simulink model "f16_hifi_euler_vTrim"  (R2020b)
settings: Solver=ode4  StartTime=0.0  StopTime=simTime  FixedStep=stepTime  RelTol=1e-3
undefined symbols (not defined in the file): data, ft, outputs, s
libraries: libAeroLookUpTables x9, aerolibconvert2 x7, lib6DOFUtilityEquations x6, libTFActuatorCalc x5, aerolibtransform2 x1, libEngineAngMomSpecs x1, libAircraftMoISpecs x1, libAircraftWeightandMassSpec x1, libAircraftWingFusalageSpecs x1, libCmdPowConversion x1, libEngineThrustCalc x1, libAtmosphereModel x1
(part 1 of 3)
settings Model: Creator=caatay  LastModifiedBy=caatay
settings DataIOCC: SaveOutput=off  SignalLogging=off  DSMLogging=off  ReturnWorkspaceOutputsName=F16_HiFi_vTrim

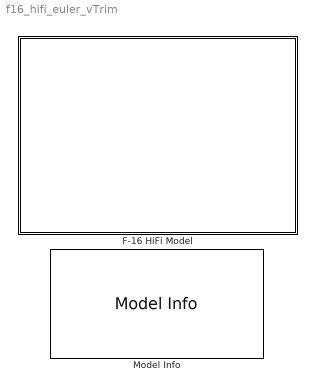
== system f16_hifi_euler_vTrim ==
  F-16 HiFi Model : Subsystem
      mask Display: image('f16-main.jpg'); % Use "Edit Image" on toolstrip to change.
  Model Info : simulink/Model-Wide Utilities/Model Info  Frame=on  DisplayStringWithTags=|  HorizontalTextAlignment=Center  LeftAlignmentValue=0.5
      | High Fidelity F-16 Just Trim Model v%<ModelVersion>
      | -------------------------------------------------------
      | Created By:  %<Creator>
      | Created at:  %<Created>
      | -------------------------------------------------------
      | Modified By: %<LastModifiedBy>
      | Modified at:  %<LastModificationDate>
      | -------------------------------------------------------

== system f16_hifi_euler_vTrim/F-16 HiFi Model ==
  Actuator Model : Subsystem
      mask Display: image('f16-actuator2.jpg'); % Use "Edit Image" on toolstrip to change.
  Aerodynamic Model : Subsystem
      mask Display: image('f16-aerodynamic.jpg'); % Use "Edit Image" on toolstrip to change.
  Aircraft Specifications : Subsystem
      mask Display: image('f16-aircraftSpec.png'); % Use "Edit Image" on toolstrip to change.
  Engine Model : Subsystem
      mask Display: image('f16-engine.jpg'); % Use "Edit Image" on toolstrip to change.
  Environment Model : Subsystem
      mask Display: image('atmosphere.jpg'); % Use "Edit Image" on toolstrip to change.
  Equation of Motion : Subsystem
      mask Display: image('f16-eom.png'); % Use "Edit Image" on toolstrip to change.
  Flight Control System & Cockpit : Subsystem
      mask Display: image('f16-cockpit.jpg'); % Use "Edit Image" on toolstrip to change.
  FlightGear Animation : libFlightGearAnimation/FlightGear Animation  Commented=on  stepTime=stepTime  mask(Animation Model - Flight Gear Animation Model){}
      mask Display: image('flightGear-logo.png'); % Use "Edit Image" on toolstrip to change.
  wires:
  Flight Control System & Cockpit/1(pilotSignal) -> [pilotCmds]
  [pilotCmds] -> Actuator Model/1(pilotCmds)
  Actuator Model/1(actSignal) -> [actSignal]
  [pilotCmds] -> Engine Model/2(pilotCmds)
  Engine Model/1(engine) -> [engine]
  Environment Model/1(atmParam) -> [atmParam]
  Environment Model/2(graParam) -> [graParam]
  [atmParam] -> Engine Model/3(atmParam)
  [atmParam] -> Flight Control System & Cockpit/2(atmParams)
  [graParam] -> Aircraft Specifications/1(graParam)
  Aircraft Specifications/1(specs) -> [acSpec]
  [actSignal] -> Aerodynamic Model/2(actSignals)
  [atmParam] -> Aerodynamic Model/3(atmParams)
  Flight Control System & Cockpit/2(stateInf) -> [states]
  [states] -> Engine Model/1(states)
  [states] -> Flight Control System & Cockpit/1(states)
  [states] -> Environment Model/1(states)
  [states] -> Aerodynamic Model/1(states)
  Aerodynamic Model/1(aeroFM) -> [aeroFM]
  [states] -> Equation of Motion/1(states)
  [graParam] -> Equation of Motion/2(graParam)
  [acSpec] -> Equation of Motion/3(acSpecs)
  [engine] -> Equation of Motion/4(engine)
  [aeroFM] -> Equation of Motion/5(aeroFM)
  Equation of Motion/2(sensorData) -> [sensorData]
  Equation of Motion/1(ders) -> [ders]
  [ders] -> Flight Control System & Cockpit/4(derivatives)
  [sensorData] -> Flight Control System & Cockpit/3(sensorData)
  [engine] -> Flight Control System & Cockpit/5(engine)
  [graParam] -> Flight Control System & Cockpit/6(gravity)
  [aeroFM] -> Flight Control System & Cockpit/7(aeroFM)
  [states] -> FlightGear Animation/1
  [sensorData] -> FlightGear Animation/2
  [actSignal] -> FlightGear Animation/3

== system f16_hifi_euler_vTrim/F-16 HiFi Model/Actuator Model ==
  In Bus Element : Inport  PortName=pilotCmds  Element=ele
  In Bus Element1 : Inport  PortName=pilotCmds  Element=ail
  In Bus Element2 : Inport  PortName=pilotCmds  Element=rud
  In Bus Element3 : Inport  PortName=pilotCmds  Element=sb
  In Bus Element4 : Inport  PortName=pilotCmds  Element=lef
  Aileron Actuator : libTFActuatorCalc/Aileron Actuator  ail=outputs.trim.controls.aileron  cmd_ail_upper_limit=21.5  cmd_ail_lower_limit=-21.5  rate_ail_upper_limit=80  rate_ail_lower_limit=-80  ail_timeCons=20.2
      settings: SourceProductName=F16 Aircraft Sub System Models
  Elevator Actuator : libTFActuatorCalc/Elevator Actuator  ele=outputs.trim.controls.elevator  cmd_ele_upper_limit=25  cmd_ele_lower_limit=-25  rate_ele_upper_limit=60  rate_ele_lower_limit=-60  ele_timeCons=20.2
      settings: SourceProductName=F16 Aircraft Sub System Models
  Leading Edge Flap Actuator : libTFActuatorCalc/Leading Edge Flap Actuator  lef=outputs.trim.controls.lef  cmd_lef_upper_limit=25  cmd_lef_lower_limit=0  rate_lef_upper_limit=25  rate_lef_lower_limit=-25  lef_timeCons=1/0.136
      settings: SourceProductName=F16 Aircraft Sub System Models
  Rudder Actuator : libTFActuatorCalc/Rudder Actuator  rud=outputs.trim.controls.rudder  cmd_rud_upper_limit=30  cmd_rud_lower_limit=-30  rate_rud_upper_limit=120  rate_rud_lower_limit=-120  rud_timeCons=20.2
      settings: SourceProductName=F16 Aircraft Sub System Models
  Speed Breaker Actuator : libTFActuatorCalc/Speed Breaker Actuator  sb=outputs.trim.controls.sb  cmd_sb_upper_limit=60  cmd_sb_lower_limit=0  rate_sb_upper_limit=60  rate_sb_lower_limit=-60  sb_timeCons=20.2
      settings: SourceProductName=F16 Aircraft Sub System Models
  Out Bus Element1 : Outport  PortName=actSignal  Element=ele
  Out Bus Element2 : Outport  PortName=actSignal  Element=ail
  Out Bus Element3 : Outport  PortName=actSignal  Element=rud
  Out Bus Element4 : Outport  PortName=actSignal  Element=sb
  Out Bus Element5 : Outport  PortName=actSignal  Element=lef
  wires:
  In Bus Element/1 -> Elevator Actuator/1
  In Bus Element1/1 -> Aileron Actuator/1
  In Bus Element2/1 -> Rudder Actuator/1
  In Bus Element3/1 -> Speed Breaker Actuator/1
  In Bus Element4/1 -> Leading Edge Flap Actuator/1
  Leading Edge Flap Actuator/1 -> Out Bus Element5/1
  Speed Breaker Actuator/1 -> Out Bus Element4/1
  Rudder Actuator/1 -> Out Bus Element3/1
  Aileron Actuator/1 -> Out Bus Element2/1
  Elevator Actuator/1 -> Out Bus Element1/1

== system f16_hifi_euler_vTrim/F-16 HiFi Model/Aerodynamic Model ==
  states : Inport
  actSignals : Inport  Port=2
  atmParams : Inport  Port=3
  Aerodynamic Look-Up Tables Interpolations : Subsystem
  Subsystem : Subsystem
  Total Coefficient Calculations : Subsystem
  aeroFM : Outport
  wires:
  actSignals/1 -> [actSignal]
  [actSignal] -> Aerodynamic Look-Up Tables Interpolations/2(actSignals)
  Aerodynamic Look-Up Tables Interpolations/1(coeffs) -> Total Coefficient Calculations/1(coeffs)
  [actSignal] -> Total Coefficient Calculations/3(actSignals)
  Total Coefficient Calculations/1(totalCoeffs) -> Subsystem/1(totalCoeffs)
  atmParams/1 -> [atmParam]
  [atmParam] -> Subsystem/3(atmParams)
  Subsystem/1(aeroFM) -> aeroFM/1
  states/1 -> [states]
  [states] -> Aerodynamic Look-Up Tables Interpolations/1(states)
  [states] -> Total Coefficient Calculations/2(states)
  [states] -> Subsystem/2(states)

== system f16_hifi_euler_vTrim/F-16 HiFi Model/Aircraft Specifications ==
  In Bus Element : Inport  PortName=graParam  Element=g_z
  Angular Momentum of Engine : libEngineAngMomSpecs/Angular Momentum of Engine  data=data
      settings: SourceProductName=F16 Aircraft Sub System Models
  Moment of Inertia Specifications : libAircraftMoISpecs/Moment of Inertia Specifications  I_xx=data.acSpec.inertia.I_xx  I_yy=data.acSpec.inertia.I_yy  I_zz=data.acSpec.inertia.I_zz  I_xz=data.acSpec.inertia.I_xz
      settings: SourceProductName=F16 Aircraft Sub System Models
  Weight of Aircraft : libAircraftWeightandMassSpec/Weight of Aircraft  G=data.acSpec.general.empWeight
      settings: SourceProductName=F16 Aircraft Sub System Models
  Wing/Aero : libAircraftWingFusalageSpecs/Wing//Aero  S=data.acSpec.wing.S  cbar=data.acSpec.wing.cbar  b=data.acSpec.wing.b  xcg=data.acSpec.fusalage.x_cg  xcg_ref=data.acSpec.fusalage.x_cg_ref
      settings: SourceProductName=F16 Aircraft Sub System Models
  Out Bus Element : Outport  PortName=specs  Element=S
  Out Bus Element1 : Outport  PortName=specs  Element=cbar
  Out Bus Element2 : Outport  PortName=specs  Element=b
  Out Bus Element3 : Outport  PortName=specs  Element=x_cg
  Out Bus Element4 : Outport  PortName=specs  Element=x_cg_ref
  Out Bus Element5 : Outport  PortName=specs  Element=h_x
  Out Bus Element6 : Outport  PortName=specs  Element=h_y
  Out Bus Element7 : Outport  PortName=specs  Element=h_z
  Out Bus Element8 : Outport  PortName=specs  Element=I_xx
  Out Bus Element9 : Outport  PortName=specs  Element=I_yy
  Out Bus Element10 : Outport  PortName=specs  Element=I_zz
  Out Bus Element11 : Outport  PortName=specs  Element=I_xz
  Out Bus Element12 : Outport  PortName=specs  Element=G
  Out Bus Element13 : Outport  PortName=specs  Element=m
  wires:
  In Bus Element/1 -> Weight of Aircraft/1
  Wing/Aero/5 -> Out Bus Element4/1
  Wing/Aero/1 -> Out Bus Element/1
  Wing/Aero/2 -> Out Bus Element1/1
  Wing/Aero/3 -> Out Bus Element2/1
  Wing/Aero/4 -> Out Bus Element3/1
  Moment of Inertia Specifications/4 -> Out Bus Element11/1
  Moment of Inertia Specifications/1 -> Out Bus Element8/1
  Moment of Inertia Specifications/2 -> Out Bus Element9/1
  Moment of Inertia Specifications/3 -> Out Bus Element10/1
  Weight of Aircraft/2 -> Out Bus Element13/1
  Weight of Aircraft/1 -> Out Bus Element12/1
  Angular Momentum of Engine/2 -> Out Bus Element6/1
  Angular Momentum of Engine/1 -> Out Bus Element5/1
  Angular Momentum of Engine/3 -> Out Bus Element7/1

== system f16_hifi_euler_vTrim/F-16 HiFi Model/Engine Model ==
  In Bus Element : Inport  PortName=states  Element=z_e
  In Bus Element1 : Inport  PortName=states  Element=power
  In Bus Element2 : Inport  Port=2  PortName=pilotCmds  Element=thrtl
  In Bus Element3 : Inport  Port=3  PortName=atmParam  Element=mach
  Throttle to Power : libCmdPowConversion/Throttle to Power
      settings: SourceProductName=F16 Aircraft Sub System Models
  Thrust Calculation : libEngineThrustCalc/Thrust Calculation
      settings: SourceProductName=F16 Aircraft Sub System Models
  Out Bus Element : Outport  PortName=engine  Element=cmdPow
  Out Bus Element1 : Outport  PortName=engine  Element=thrust
  wires:
  In Bus Element/1 -> Thrust Calculation/1
  In Bus Element1/1 -> Thrust Calculation/3
  In Bus Element2/1 -> Throttle to Power/1
  In Bus Element3/1 -> Thrust Calculation/2
  Throttle to Power/1 -> Out Bus Element/1
  Thrust Calculation/1 -> Out Bus Element1/1

== system f16_hifi_euler_vTrim/F-16 HiFi Model/Environment Model ==
  In Bus Element : Inport  PortName=states  Element=tas
  In Bus Element1 : Inport  PortName=states  Element=z_e
  In Bus Element2 : Inport  PortName=states  Element=z_e
  In Bus Element4 : Inport  PortName=states  Element=x_e
  In Bus Element3 : Inport  PortName=states  Element=y_e
  In Bus Element5 : Inport  PortName=states  Element=lat
  In Bus Element10 : Inport  PortName=states  Element=long
  Atmosphere Model : libAtmosphereModel/Atmosphere Model  lapse_rate=0.703e-5  rho_0=2.377e-3  k=1.4
      settings: SourceProductName=F16 Aircraft Sub System Models
  WGS84 Gravity Model : libGravityModel/WGS84 Gravity Model  h_0=0  a=6378137  b=6356752  w_e=[0; 0; 7.29115e-05]  GM=3986004.418e8  R_e=6378137  J_2=1.082626684e-3
      settings: SourceProductName=F16 Aircraft Sub System Models
  Out Bus Element : Outport  PortName=atmParam  Element=temp
  Out Bus Element1 : Outport  PortName=atmParam  Element=rho
  Out Bus Element2 : Outport  PortName=atmParam  Element=a
  Out Bus Element3 : Outport  PortName=atmParam  Element=mach
  Out Bus Element4 : Outport  PortName=atmParam  Element=qbar
  Out Bus Element5 : Outport  PortName=atmParam  Element=pSta
  Out Bus Element6 : Outport  Port=2  PortName=graParam  Element=g_x
  Out Bus Element7 : Outport  Port=2  PortName=graParam  Element=g_y
  Out Bus Element8 : Outport  Port=2  PortName=graParam  Element=g_z
  wires:
  In Bus Element10/1 -> WGS84 Gravity Model/5
  In Bus Element4/1 -> WGS84 Gravity Model/1
  In Bus Element2/1 -> WGS84 Gravity Model/3
  In Bus Element1/1 -> Atmosphere Model/2
  In Bus Element/1 -> Atmosphere Model/1
  In Bus Element3/1 -> WGS84 Gravity Model/2
  In Bus Element5/1 -> WGS84 Gravity Model/4
  Atmosphere Model/1 -> Out Bus Element/1
  Atmosphere Model/2 -> Out Bus Element1/1
  Atmosphere Model/3 -> Out Bus Element2/1
  Atmosphere Model/4 -> Out Bus Element3/1
  Atmosphere Model/5 -> Out Bus Element4/1
  Atmosphere Model/6 -> Out Bus Element5/1
  WGS84 Gravity Model/3 -> Out Bus Element8/1
  WGS84 Gravity Model/2 -> Out Bus Element7/1
  WGS84 Gravity Model/1 -> Out Bus Element6/1

== system f16_hifi_euler_vTrim/F-16 HiFi Model/Equation of Motion ==
  states : Inport
  graParam : Inport  Port=2
  acSpecs : Inport  Port=3
  engine : Inport  Port=4
  aeroFM : Inport  Port=5
  Derivative Equations : Subsystem
  Utility Functions : Subsystem
  ders : Outport
  sensorData : Outport  Port=2
  wires:
  [states] -> Utility Functions/1(states)
  states/1 -> [states]
  graParam/1 -> [graParam]
  [graParam] -> Utility Functions/2(graParam)
  [ders] -> Utility Functions/3(ders)
  Utility Functions/1(sensorData) -> sensorData/1, [sensorData]
  [sensorData] -> Derivative Equations/6(sensorData)
  [states] -> Derivative Equations/1(states)
  [graParam] -> Derivative Equations/4(graParam)
  [aeroFM] -> Derivative Equations/2(aeroFM)
  [engine] -> Derivative Equations/3(engine)
  [acSpec] -> Derivative Equations/5(acSpecs)
  aeroFM/1 -> [aeroFM]
  engine/1 -> [engine]
  acSpecs/1 -> [acSpec]
  Derivative Equations/1(ders) -> ders/1, [ders]

== system f16_hifi_euler_vTrim/F-16 HiFi Model/Flight Control System & Cockpit ==
  states : Inport
  atmParams : Inport  Port=2
  sensorData : Inport  Port=3
  derivatives : Inport  Port=4
  engine : Inport  Port=5
  gravity : Inport  Port=6
  aeroFM : Inport  Port=7
  Bus Creator : BusCreator  Inputs=6
  Bus Selector : BusSelector  OutputSignals=alpha
  Bus Selector1 : BusSelector  OutputSignals=qbar,pSta
  Data Storeage : libResultDataStorer/Data Storeage
      settings: SourceProductName=F16 Aircraft Sub System Models
  Integrator : libIntegratorModel/Integrator  outputs=outputs
      settings: SourceProductName=F16 Aircraft Sub System Models
  Leading Edge Flap Model : libLeadingEdgeFlapDefCalc/Leading Edge Flap Model  initAlphaDeg=-outputs.trim.states.alpha*180/pi
      settings: SourceProductName=F16 Aircraft Sub System Models
  Scopes : Subsystem  mask(Flight Control System - Simulation Scopes){}
      mask help: Simulation Result grapher to obtain whole simulation results.
      mask Help:
      | This block integrate state derivative to state variables.
      | -------------------------------------------------------------------------------------------------------------------------------------------------
      | Inputs of this block set are:
      | 	states: Information of state variables.
      | 	sensorData: Information of sensor data.
      | 	engine: Information of engine.
      | 	atm: Information of atmosphere parameters.
      | 	gravity: Information of gravity Parameters.
      | 	commands: Information of pilot commands and flight surfaces
      | -------------------------------------------------------------------------------------------------------------------------------------------------
      | For question: "cagataysahin44@gmail.com"
      mask Display:
      | port_label('input',1,'Inf_{states}','texmode','on');
      | port_label('input',2,'Inf_{sensor}','texmode','on');
      | port_label('input',3,'Inf_{engine}','texmode','on');
      | port_label('input',4,'Inf_{atm}','texmode','on');
      | port_label('input',5,'Inf_{gravity}','texmode','on');
      | port_label('input',6,'Inf_{commands}','texmode','on');
  Trim Conditions : libControlTrimInputs/Trim Conditions  throttle=outputs.trim.controls.throttle  elevator=outputs.trim.controls.elevator  aileron=outputs.trim.controls.aileron  rudder=outputs.trim.controls.rudder  sb=outputs.trim.controls.sb
      settings: SourceProductName=F16 Aircraft Sub System Models
  Out Bus Element : Outport  PortName=pilotSignal  Element=thrtl
  Out Bus Element1 : Outport  PortName=pilotSignal  Element=ele
  Out Bus Element2 : Outport  PortName=pilotSignal  Element=ail
  Out Bus Element3 : Outport  PortName=pilotSignal  Element=rud
  Out Bus Element4 : Outport  PortName=pilotSignal  Element=sb
  Out Bus Element5 : Outport  PortName=pilotSignal  Element=lef
  stateInf : Outport  Port=2
  wires:
  Trim Conditions/4 -> Bus Creator/4, Out Bus Element3/1  "rud"
  Trim Conditions/3 -> Bus Creator/3, Out Bus Element2/1  "ail"
  Trim Conditions/1 -> Bus Creator/1, Out Bus Element/1  "thrtl"
  Leading Edge Flap Model/1 -> Bus Creator/6, Out Bus Element5/1  "lef"
  Integrator/1 -> stateInf/1
  derivatives/1 -> [ders]
  sensorData/1 -> [sensorData]
  [sensorData] -> Integrator/2
  [ders] -> Integrator/1
  [sensorData] -> Scopes/2(sensorData)
  atmParams/1 -> [atmParam]
  states/1 -> [states]
  engine/1 -> [engine]
  gravity/1 -> [graParam]
  [states] -> Scopes/1(states)
  [atmParam] -> Scopes/4(atmParam)
  [engine] -> Scopes/3(engine)
  [graParam] -> Scopes/5(graParam)
  [states] -> Bus Selector/1
  Bus Selector/1 -> Leading Edge Flap Model/1  "<alpha>"
  [atmParam] -> Bus Selector1/1
  Bus Selector1/1 -> Leading Edge Flap Model/2  "<qbar>"
  Bus Selector1/2 -> Leading Edge Flap Model/3  "<pSta>"
  Trim Conditions/2 -> Bus Creator/2, Out Bus Element1/1  "ele"
  Trim Conditions/5 -> Bus Creator/5, Out Bus Element4/1  "sb"
  Bus Creator/1 -> [pilotCmds]
  [pilotCmds] -> Scopes/6(pilotSignals)
  aeroFM/1 -> [aeroFM]
  [aeroFM] -> Data Storeage/7
  [pilotCmds] -> Data Storeage/6
  [graParam] -> Data Storeage/5
  [atmParam] -> Data Storeage/4
  [engine] -> Data Storeage/3
  [sensorData] -> Data Storeage/2
  [states] -> Data Storeage/1

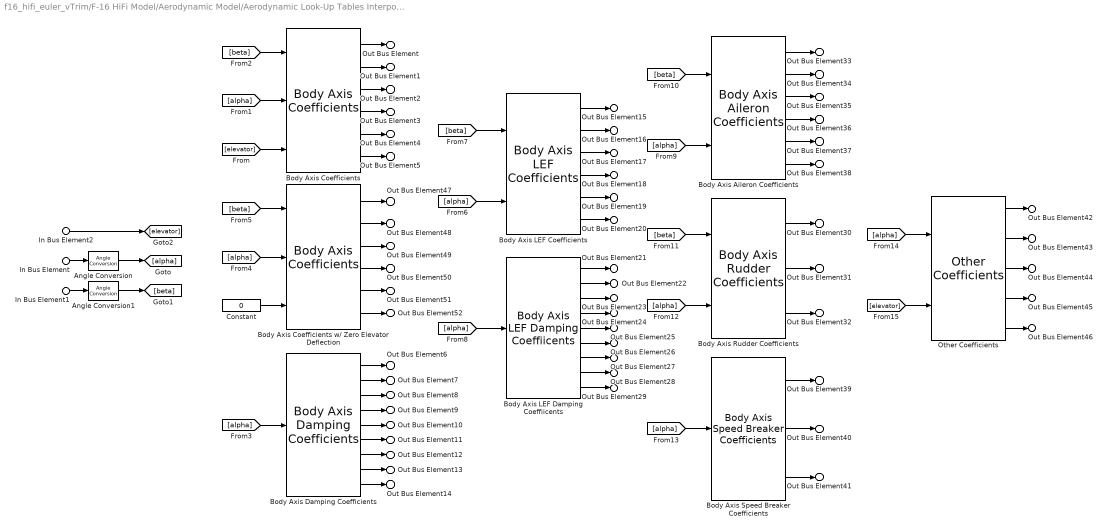
== system f16_hifi_euler_vTrim/F-16 HiFi Model/Aerodynamic Model/Aerodynamic Look-Up Tables Interpolations ==
  In Bus Element : Inport  PortName=states  Element=alpha
  In Bus Element1 : Inport  PortName=states  Element=beta
  In Bus Element2 : Inport  Port=2  PortName=actSignals  Element=ele
  Angle Conversion : aerolibconvert2/Angle Conversion  IU=rad  OU=deg
  Angle Conversion1 : aerolibconvert2/Angle Conversion  IU=rad  OU=deg
  Body Axis Aileron Coefficients : libAeroLookUpTables/Body Axis Aileron Coefficients  data=data
      settings: SourceProductName=F16 Aircraft Sub System Models
  Body Axis Coefficients : libAeroLookUpTables/Body Axis Coefficients  data=data
      settings: SourceProductName=F16 Aircraft Sub System Models
  Body Axis Coefficients w/ Zero Elevator Deflection : libAeroLookUpTables/Body Axis Coefficients  data=data
      settings: SourceProductName=F16 Aircraft Sub System Models
  Body Axis Damping Coefficients : libAeroLookUpTables/Body Axis Damping Coefficients  data=data
      settings: SourceProductName=F16 Aircraft Sub System Models
  Body Axis LEF Damping Coeffiicents : libAeroLookUpTables/Body Axis LEF  Damping Coeffiicents  data=data
      settings: SourceProductName=F16 Aircraft Sub System Models
  Body Axis LEF Coefficients : libAeroLookUpTables/Body Axis LEF Coefficients  data=data
      settings: SourceProductName=F16 Aircraft Sub System Models
  Body Axis Rudder Coefficients : libAeroLookUpTables/Body Axis Rudder Coefficients  data=data
      settings: SourceProductName=F16 Aircraft Sub System Models
  Body Axis Speed Breaker Coefficients : libAeroLookUpTables/Body Axis Speed Breaker Coefficients  data=data
      settings: SourceProductName=F16 Aircraft Sub System Models
  Constant : Constant  Value=0
  Other Coefficients : libAeroLookUpTables/Other Coefficients  data=data
      settings: SourceProductName=F16 Aircraft Sub System Models
  Out Bus Element : Outport  PortName=coeffs  Element=Cx
  Out Bus Element1 : Outport  PortName=coeffs  Element=Cy
  Out Bus Element2 : Outport  PortName=coeffs  Element=Cz
  Out Bus Element3 : Outport  PortName=coeffs  Element=Cl
  Out Bus Element4 : Outport  PortName=coeffs  Element=Cm
  Out Bus Element5 : Outport  PortName=coeffs  Element=Cn
  Out Bus Element47 : Outport  PortName=coeffs  Element=Cx0
  Out Bus Element48 : Outport  PortName=coeffs  Element=Cy0
  Out Bus Element49 : Outport  PortName=coeffs  Element=Cz0
  Out Bus Element50 : Outport  PortName=coeffs  Element=Cl0
  Out Bus Element51 : Outport  PortName=coeffs  Element=Cm0
  Out Bus Element52 : Outport  PortName=coeffs  Element=Cn0
  Out Bus Element6 : Outport  PortName=coeffs  Element=Cxq
  Out Bus Element7 : Outport  PortName=coeffs  Element=Cyp
  Out Bus Element8 : Outport  PortName=coeffs  Element=Cyr
  Out Bus Element9 : Outport  PortName=coeffs  Element=Czq
  Out Bus Element10 : Outport  PortName=coeffs  Element=Clp
  Out Bus Element11 : Outport  PortName=coeffs  Element=Clr
  Out Bus Element12 : Outport  PortName=coeffs  Element=Cmq
  Out Bus Element13 : Outport  PortName=coeffs  Element=Cnp
  Out Bus Element14 : Outport  PortName=coeffs  Element=Cnr
  Out Bus Element15 : Outport  PortName=coeffs  Element=Cxlef
  Out Bus Element16 : Outport  PortName=coeffs  Element=Cylef
  Out Bus Element17 : Outport  PortName=coeffs  Element=Czlef
  Out Bus Element18 : Outport  PortName=coeffs  Element=Cllef
  Out Bus Element19 : Outport  PortName=coeffs  Element=Cmlef
  Out Bus Element20 : Outport  PortName=coeffs  Element=Cnlef
  Out Bus Element21 : Outport  PortName=coeffs  Element=Cxqlef
  Out Bus Element22 : Outport  PortName=coeffs  Element=Cyplef
  Out Bus Element23 : Outport  PortName=coeffs  Element=Cyrlef
  Out Bus Element24 : Outport  PortName=coeffs  Element=Czqlef
  Out Bus Element25 : Outport  PortName=coeffs  Element=Clplef
  Out Bus Element26 : Outport  PortName=coeffs  Element=Clrlef
  Out Bus Element27 : Outport  PortName=coeffs  Element=Cmqlef
  Out Bus Element28 : Outport  PortName=coeffs  Element=Cnplef
  Out Bus Element29 : Outport  PortName=coeffs  Element=Cnrlef
  Out Bus Element33 : Outport  PortName=coeffs  Element=Cyail
  Out Bus Element34 : Outport  PortName=coeffs  Element=Cyaillef
  Out Bus Element35 : Outport  PortName=coeffs  Element=Clail
  Out Bus Element36 : Outport  PortName=coeffs  Element=Claillef
  Out Bus Element37 : Outport  PortName=coeffs  Element=Cnail
  Out Bus Element38 : Outport  PortName=coeffs  Element=Cnaillef
  Out Bus Element30 : Outport  PortName=coeffs  Element=Cyrud
  Out Bus Element31 : Outport  PortName=coeffs  Element=Clrud
  Out Bus Element32 : Outport  PortName=coeffs  Element=Cnrud
  Out Bus Element39 : Outport  PortName=coeffs  Element=Cxsb
  Out Bus Element40 : Outport  PortName=coeffs  Element=Czsb
  Out Bus Element41 : Outport  PortName=coeffs  Element=Cmsb
  Out Bus Element42 : Outport  PortName=coeffs  Element=Clbeta
  Out Bus Element43 : Outport  PortName=coeffs  Element=Cnbeta
  Out Bus Element44 : Outport  PortName=coeffs  Element=Cmdiff
  Out Bus Element45 : Outport  PortName=coeffs  Element=Cmeta
  Out Bus Element46 : Outport  PortName=coeffs  Element=Cmds
  wires:
  Angle Conversion1/1 -> [beta]
  In Bus Element2/1 -> [elevator]
  Angle Conversion/1 -> [alpha]
  In Bus Element1/1 -> Angle Conversion1/1
  In Bus Element/1 -> Angle Conversion/1
  [elevator] -> Body Axis Coefficients/3
  [alpha] -> Body Axis Coefficients/2
  [beta] -> Body Axis Coefficients/1
  Body Axis Coefficients/6 -> Out Bus Element5/1
  Body Axis Coefficients/5 -> Out Bus Element4/1
  Body Axis Coefficients/2 -> Out Bus Element1/1
  Body Axis Coefficients/3 -> Out Bus Element2/1
  Body Axis Coefficients/1 -> Out Bus Element/1
  Body Axis Coefficients/4 -> Out Bus Element3/1
  Body Axis Coefficients w/ Zero Elevator Deflection/2 -> Out Bus Element48/1
  Body Axis Coefficients w/ Zero Elevator Deflection/5 -> Out Bus Element51/1
  Body Axis Coefficients w/ Zero Elevator Deflection/6 -> Out Bus Element52/1
  Body Axis Coefficients w/ Zero Elevator Deflection/3 -> Out Bus Element49/1
  Body Axis Coefficients w/ Zero Elevator Deflection/4 -> Out Bus Element50/1
  [beta] -> Body Axis Coefficients w/ Zero Elevator Deflection/1
  [alpha] -> Body Axis Coefficients w/ Zero Elevator Deflection/2
  Body Axis Coefficients w/ Zero Elevator Deflection/1 -> Out Bus Element47/1
  Constant/1 -> Body Axis Coefficients w/ Zero Elevator Deflection/3
  [alpha] -> Body Axis Damping Coefficients/1
  Body Axis Damping Coefficients/7 -> Out Bus Element12/1
  Body Axis Damping Coefficients/3 -> Out Bus Element8/1
  Body Axis Damping Coefficients/5 -> Out Bus Element10/1
  Body Axis Damping Coefficients/6 -> Out Bus Element11/1
  Body Axis Damping Coefficients/8 -> Out Bus Element13/1
  Body Axis Damping Coefficients/9 -> Out Bus Element14/1
  Body Axis Damping Coefficients/1 -> Out Bus Element6/1
  Body Axis Damping Coefficients/2 -> Out Bus Element7/1
  Body Axis Damping Coefficients/4 -> Out Bus Element9/1
  [alpha] -> Body Axis LEF Coefficients/2
  [beta] -> Body Axis LEF Coefficients/1
  Body Axis LEF Coefficients/2 -> Out Bus Element16/1
  Body Axis LEF Coefficients/4 -> Out Bus Element18/1
  Body Axis LEF Coefficients/1 -> Out Bus Element15/1
  Body Axis LEF Coefficients/6 -> Out Bus Element20/1
  Body Axis LEF Coefficients/3 -> Out Bus Element17/1
  Body Axis LEF Coefficients/5 -> Out Bus Element19/1
  [alpha] -> Body Axis LEF Damping Coeffiicents/1
  Body Axis LEF Damping Coeffiicents/6 -> Out Bus Element26/1
  Body Axis LEF Damping Coeffiicents/4 -> Out Bus Element24/1
  Body Axis LEF Damping Coeffiicents/2 -> Out Bus Element22/1
  Body Axis LEF Damping Coeffiicents/9 -> Out Bus Element29/1
  Body Axis LEF Damping Coeffiicents/5 -> Out Bus Element25/1
  Body Axis LEF Damping Coeffiicents/1 -> Out Bus Element21/1
  Body Axis LEF Damping Coeffiicents/7 -> Out Bus Element27/1
  Body Axis LEF Damping Coeffiicents/8 -> Out Bus Element28/1
  Body Axis LEF Damping Coeffiicents/3 -> Out Bus Element23/1
  [beta] -> Body Axis Aileron Coefficients/1
  [alpha] -> Body Axis Aileron Coefficients/2
  Body Axis Aileron Coefficients/4 -> Out Bus Element36/1
  Body Axis Aileron Coefficients/3 -> Out Bus Element35/1
  Body Axis Aileron Coefficients/5 -> Out Bus Element37/1
  Body Axis Aileron Coefficients/1 -> Out Bus Element33/1
  Body Axis Aileron Coefficients/6 -> Out Bus Element38/1
  Body Axis Aileron Coefficients/2 -> Out Bus Element34/1
  [alpha] -> Body Axis Rudder Coefficients/2
  Body Axis Rudder Coefficients/3 -> Out Bus Element32/1
  Body Axis Rudder Coefficients/1 -> Out Bus Element30/1
  Body Axis Rudder Coefficients/2 -> Out Bus Element31/1
  [alpha] -> Body Axis Speed Breaker Coefficients/1
  Body Axis Speed Breaker Coefficients/3 -> Out Bus Element41/1
  Body Axis Speed Breaker Coefficients/2 -> Out Bus Element40/1
  Body Axis Speed Breaker Coefficients/1 -> Out Bus Element39/1
  [alpha] -> Other Coefficients/1
  [elevator] -> Other Coefficients/2
  Other Coefficients/1 -> Out Bus Element42/1
  Other Coefficients/2 -> Out Bus Element43/1
  Other Coefficients/3 -> Out Bus Element44/1
  Other Coefficients/4 -> Out Bus Element45/1
  Other Coefficients/5 -> Out Bus Element46/1
  [beta] -> Body Axis Rudder Coefficients/1

== system f16_hifi_euler_vTrim/F-16 HiFi Model/Aerodynamic Model/Subsystem ==
  In Bus Element : Inport  PortName=totalCoeffs  Element=Cl
  In Bus Element3 : Inport  PortName=totalCoeffs  Element=Cx
  In Bus Element4 : Inport  PortName=totalCoeffs  Element=Cy
  In Bus Element5 : Inport  PortName=totalCoeffs  Element=Cz
  In Bus Element1 : Inport  PortName=totalCoeffs  Element=Cm
  In Bus Element10 : Inport  PortName=totalCoeffs  Element=Cn
  In Bus Element6 : Inport  Port=2  PortName=states  Element=alpha
  In Bus Element7 : Inport  Port=2  PortName=states  Element=beta
  In Bus Element8 : Inport  Port=3  PortName=atmParams  Element=qbar
  In Bus Element9 : Inport  Port=3  PortName=atmParams  Element=qbar
  Aerodynamic Forces : Subsystem  mask(Aerodynamic Model -> Aerodynamic Forces and Moment Calculation -> Aerodynamic Force Calculation){S=data.acSpec.wing.S}
      mask prompts: S "Wing Aera"
      mask help: Aerodynamic Force calculation block calculates body axis aerodynamic forces with using atmosphere and aircraft wing information.
      mask Help:
      | This block can calculate body axis aerodynamic forces with using atmosphere and aircraft wing information.
      | Just calculate body axis forces.
      | -------------------------------------------------------------------------------------------------------------------------------------------------
      | Inputs of this block:
      | 	C_{i}: Aerodynamic total ceofficients.
      | 	qbar: Dynamic Pressure in [lb/ft^2].
      | 	S: Wing Reference Area [ft^2].
      | Outputs of this block:
      | 	F_{i}: Body axis forces in i axis.
      | -------------------------------------------------------------------------------------------------------------------------------------------------
      | 	- Equations that in this block can be found in Steven's textbook. This textbook is in "literature" subfolder.
      | 	- for question: "cagataysahin44@gmail.com".
      mask Display:
      | port_label('input',1,'C_{i}','texmode','on');
      | port_label('input',2,'qbar','texmode','on');
      | port_label('input',3,'\alpha','texmode','on');
      | port_label('input',4,'\beta','texmode','on');
      | 
      | port_label('output',1,'F_{x}','texmode','on');
      | port_label('output',2,'F_{y}','texmode','on');
      | port_label('output',3,'F_{z}','texmode','on');
      | port_label('output',4,'D','texmode','on');
      | port_label('output',5,'C','texmode','on');
      | port_label('output',6,'L','texmode','on');
  Aerodynamic Moments : Subsystem  mask(Aerodynamic Model -> Aerodynamic Forces and Moment Calculation -> Aerodynamic Moment Calculation){S=data.acSpec.wing.S, b=data.acSpec.wing.b, cbar=data.acSpec.wing.cbar}
      mask prompts: S "Wing Area"; b "Wing Span"; cbar "Mean Aerodynamic Chord"
      mask help: Aerodynamic moment calculation block calculates body axis aerodynamic forces with using atmosphere and aircraft wing information.
      mask Help:
      | This block can calculate body axis aerodynamic moments with using atmosphere and aircraft wing information.
      | -------------------------------------------------------------------------------------------------------------------------------------------------
      | Inputs of this block:
      | 	C_{i}: Aerodynamic total ceofficients.
      | 	qbar: Dynamic Pressure in [lb/ft^2].
      | 	S: Wing Reference Area [ft^2].
      | 	b: Wing Span [ft].
      | 	cbar: Mean Aerodynamic Chord [ft].
      | Outputs of this block:
      | 	M_{i}: Body axis moments in i axis.
      | -------------------------------------------------------------------------------------------------------------------------------------------------
      | 	- Equations that in this block can be found in Steven's textbook. This textbook is in "literature" subfolder.
      | 	- for question: "cagataysahin44@gmail.com".
      mask Display:
      | port_label('input',1,'C_{i}','texmode','on');
      | port_label('input',2,'qbar','texmode','on');
      | 
      | port_label('output',1,'M_{l}','texmode','on');
      | port_label('output',2,'M_{m}','texmode','on');
      | port_label('output',3,'M_{n}','texmode','on');
  Mux : Mux  Inputs=3
  Mux1 : Mux  Inputs=3
  Out Bus Element : Outport  PortName=aeroFM  Element=X
  Out Bus Element1 : Outport  PortName=aeroFM  Element=Y
  Out Bus Element2 : Outport  PortName=aeroFM  Element=Z
  Out Bus Element3 : Outport  PortName=aeroFM  Element=drag
  Out Bus Element4 : Outport  PortName=aeroFM  Element=side
  Out Bus Element5 : Outport  PortName=aeroFM  Element=lift
  Out Bus Element6 : Outport  PortName=aeroFM  Element=L
  Out Bus Element7 : Outport  PortName=aeroFM  Element=M
  Out Bus Element8 : Outport  PortName=aeroFM  Element=N
  wires:
  Aerodynamic Forces/6(L) -> Out Bus Element5/1
  In Bus Element/1 -> Mux/1
  Aerodynamic Moments/2(Mm) -> Out Bus Element7/1
  Aerodynamic Moments/1(Ml) -> Out Bus Element6/1
  Aerodynamic Forces/1(Fx) -> Out Bus Element/1
  Mux/1 -> Aerodynamic Moments/1(C_i)
  Mux1/1 -> Aerodynamic Forces/1(C_i)
  In Bus Element3/1 -> Mux1/1
  In Bus Element4/1 -> Mux1/2
  In Bus Element9/1 -> Aerodynamic Moments/2(qbar)
  Aerodynamic Forces/3(Fz) -> Out Bus Element2/1
  In Bus Element1/1 -> Mux/2
  In Bus Element10/1 -> Mux/3
  In Bus Element7/1 -> Aerodynamic Forces/4(beta)
  Aerodynamic Moments/3(Mn) -> Out Bus Element8/1
  In Bus Element8/1 -> Aerodynamic Forces/2(qbar)
  In Bus Element6/1 -> Aerodynamic Forces/3(alpha)
  In Bus Element5/1 -> Mux1/3
  Aerodynamic Forces/4(D) -> Out Bus Element3/1
  Aerodynamic Forces/2(Fy) -> Out Bus Element1/1
  Aerodynamic Forces/5(C) -> Out Bus Element4/1
